simulink model "AV_homo_traffic"  (R2020b)
settings: Solver=FixedStepAuto  StartTime=0.0  StopTime=3600  FixedStep=0.02  RelTol=1e-3
model workspace (MAT data in the model file):
  P_a_x = [-10 0 10]
  P_a_y = [-12.8017053517 0 14.85382]
  P_v_x = [-100 0 100]
  P_v_y = [-10.4028259584 0 12.0704]
  Range_Sensor = 250
  Set_Speeds = [50 100 150]
  a_max_x = [0 5 20 50]
  a_max_y = [7.811082 7.811082 3.905541 3.905541]
  a_min_x = [-1 0 0.0001 5 20 50]
  a_min_y = [0 0 -5 -5 -3.5 -3.5]
  cycle_dovt = [0 0 0 0 0 0 0 0 0 0 0 0 ... (21081 elements, 1x21081)]
  cycle_t = [0 0.05 0.1 0.15 0.2 0.25 0.3 0.35 0.4 0.45 0.5 0.55 ... (21361 elements, 1x21361)]
  cycle_type = [3 3 3 3 3 3 3 3 3 3 3 3 ... (21081 elements, 1x21081)]
  cycle_v = [0 0 0 0 0 0 0 0 0 0 0 0 ... (21361 elements, 1x21361)]
  cycle_x = [0 0 0 0 0 0 0 0 0 0 0 0 ... (21361 elements, 1x21361)]
  cycle_xx = [0 9.74820143885e-05 0.000573141486811 0.0017757793765 0.00401894484412 0.0075809352518 0.0127047961631 0.0195983213429 0.0284340527578 0.0393492805755 0.0524460431655 0.0677911270983 ... (21081 elements, 1x21081)]
  d0 = 2
  j_min_x = [0 5 20 50]
  j_min_y = [-8.608244 -8.608244 -4.304122 -4.304122]
  ovt_tol = 11.163335
  set_speeds = [50 100 137.38231]
  t_delta_traf = 10
  t_sensor = 0.2
  t_set = 0.651096
libraries: simulink x6
(part 1 of 2)
settings Model: PauseTimes=1  OrderedModelArguments=off  Creator=duanx  LastModifiedBy=duanx
settings DataIOCC: SaveOutput=off

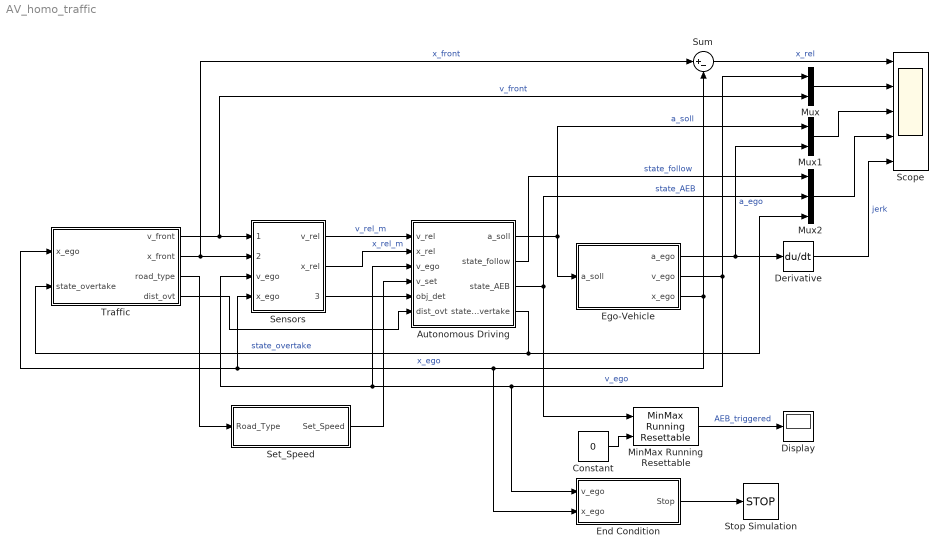
== system AV_homo_traffic ==
  Autonomous Driving : Subsystem
  Constant : Constant  Value=0
  Derivative : Derivative
  Display : Display
  Ego-Vehicle : Subsystem
  End Condition : Subsystem
  MinMax Running Resettable : simulink/Math Operations/MinMax Running Resettable  Function=max  vinit=0.0
  Mux : Mux  Inputs=2
  Mux1 : Mux  Inputs=2
  Mux2 : Mux  Inputs=3
  Scope : Scope  NumInputPorts=5
  Sensors : Subsystem
  Set_Speed : Subsystem
  Stop Simulation : Stop
  Sum : Sum  Inputs=|+-
  Traffic : Subsystem
  wires:
  Sum/1 -> Scope/1  "x_rel"
  Constant/1 -> MinMax Running Resettable/2
  Autonomous Driving/1(a_soll) -> Ego-Vehicle/1(a_soll), Mux1/1  "a_soll"
  Traffic/2(x_front) -> Sum/1, Sensors/2(x_front)  "x_front"
  Mux1/1 -> Scope/3
  Derivative/1 -> Scope/5  "jerk"
  Mux/1 -> Scope/2
  Ego-Vehicle/1(a_ego) -> Mux1/2, Derivative/1  "a_ego"
  Mux2/1 -> Scope/4
  Sensors/2(x_rel) -> Autonomous Driving/2(x_rel)  "x_rel_m"
  MinMax Running Resettable/1 -> Display/1  "AEB_triggered"
  Autonomous Driving/3(state_AEB) -> MinMax Running Resettable/1, Mux2/2  "state_AEB"
  Ego-Vehicle/3(x_ego) -> End Condition/2(x_ego), Sensors/4(x_ego), Traffic/1(x_ego), Sum/2  "x_ego"
  Autonomous Driving/2(state_follow) -> Mux2/1  "state_follow"
  Set_Speed/1(Set_Speed) -> Autonomous Driving/4(v_set)
  Sensors/1(v_rel) -> Autonomous Driving/1(v_rel)  "v_rel_m"
  Ego-Vehicle/2(v_ego) -> End Condition/1(v_ego), Sensors/3(v_ego), Autonomous Driving/3(v_ego), Mux/1  "v_ego"
  Sensors/3(Obj_det) -> Autonomous Driving/5(obj_det)
  Traffic/1(v_front) -> Mux/2, Sensors/1(v_front)  "v_front"
  Traffic/3(road_type) -> Set_Speed/1(Road_Type)
  Autonomous Driving/4(state_overtake) -> Traffic/2(state_overtake), Mux2/3  "state_overtake"
  Traffic/4(dist_ovt) -> Autonomous Driving/6(dist_ovt)
  End Condition/1(Stop) -> Stop Simulation/1
